simulink model "ConSys_A1"  (Simulink 8.3)
settings: Solver=ode3  StartTime=0.0  StopTime=Time(end)  FixedStep=Ts  RelTol=1e-3
values from neighbouring files (symbols this model uses):
  d = r*h    (= 1.6)    [StartUp_A1.m]
  d0 = d*h    (= 0.0032)    [StartUp_A1.m]
  h = 0.002    [StartUp_A1.m]
  Ka = diag([ 3  20  20  150  355  520])    [StartUp_A1.m]
  Kd = diag([ 3   5  25  100   15 1050])    [StartUp_A1.m]
  Ki = diag([35 555 810 7410 1850 5815])    [StartUp_A1.m]
  Kp = diag([55 180 350 1960  680 4450])    [StartUp_A1.m]
  r = 800    [StartUp_A1.m]
  TD = ss(Atd,Btd,Ctd,Dtd,Ts)    [StartUp_A1.m]
  Ts = 1/200    (= 0.005)    [StartUp_A1.m]
undefined symbols (not defined in the file or in its folder): DiscIntNeverNeededParam
undefined symbols (not defined in the file): ADAMS_cwd, ADAMS_exec, ADAMS_host, ADAMS_init, ADAMS_inputs, ADAMS_outputs, ADAMS_prefix, ADAMS_static, ADAMS_sysdir
libraries: cstblocks x6
(part 3 of 9)

== matlab function A/MATLAB Function 5 ==
  data: q input double; M55 output double; M56 output double
function [M55,M56] = M5(q)
%#codegen
Th1=q(1,1); Th2=q(2,1); Th3=q(3,1);
Th4=q(4,1); Th5=q(5,1); Th6=q(6,1);
M55=2.9736e-6*sin(Th6)^2 + 0.0075895;
M56=(0.5*(sin(Th2 + Th3)*cos(Th5) + cos(Th2 + Th3)*cos(Th4)*sin(Th5))*(0.01294*sin(Th5)*(sin(Th1)*sin(Th4) - 1.0*sin(Th2 + Th3)*cos(Th1)*cos(Th4)) + 0.00023*sin(Th6)*(cos(Th4)*sin(Th1) + sin(Th2 + Th3)*cos(Th1)*sin(Th4)) + 0.00023*cos(Th6)*(cos(Th5)*(sin(Th1)*sin(Th4) - 1.0*sin(Th2 + Th3)*cos(Th1)*cos(Th4)) - 1.0*cos(Th2 + Th3)*cos(Th1)*sin(Th5)) + 0.01294*cos(Th2 + Th3)*cos(Th1)*cos(Th5)) + 0.5*(sin(Th5)*(sin(Th1)*sin(Th4) - 1.0*sin(Th2 + Th3)*cos(Th1)*cos(Th4)) + cos(Th2 + Th3)*cos(Th1)*cos(Th5))*(0.00023*cos(Th6)*(sin(Th2 + Th3)*sin(Th5) - 1.0*cos(Th2 + Th3)*cos(Th4)*cos(Th5)) - 0.01294*sin(Th2 + Th3)*cos(Th5) - 0.01294*cos(Th2 + Th3)*cos(Th4)*sin(Th5) + 0.00023*cos(Th2 + Th3)*sin(Th4)*sin(Th6)))*(0.05206*cos(Th2 + Th3)*sin(Th1)*sin(Th5) + 0.05206*cos(Th1)*cos(Th5)*sin(Th4) - 0.00023*cos(Th2 + Th3)*cos(Th5)*cos(Th6)*sin(Th1) + 0.05206*sin(Th2 + Th3)*cos(Th4)*cos(Th5)*sin(Th1) + 0.00023*cos(Th1)*cos(Th6)*sin(Th4)*sin(Th5) + 0.00023*sin(Th2 + Th3)*cos(Th4)*cos(Th6)*sin(Th1)*sin(Th5)) + (0.000115*cos(Th2 + Th3)*cos(Th6)*sin(Th4) - 0.000115*sin(Th2 + Th3)*sin(Th5)*sin(Th6) + 0.000115*cos(Th2 + Th3)*cos(Th4)*cos(Th5)*sin(Th6))*(0.05206*cos(Th2 + Th3)*cos(Th4)*cos(Th5) - 0.05206*sin(Th2 + Th3)*sin(Th5) + 0.00023*sin(Th2 + Th3)*cos(Th5)*cos(Th6) + 0.00023*cos(Th2 + Th3)*cos(Th4)*cos(Th6)*sin(Th5)) + (sin(Th5)*(cos(Th1)*sin(Th4) + sin(Th2 + Th3)*cos(Th4)*sin(Th1)) - 1.0*cos(Th2 + Th3)*cos(Th5)*sin(Th1))*((cos(Th1)*cos(Th4) - 1.0*sin(Th2 + Th3)*sin(Th1)*sin(Th4))*((0.00104*cos(Th6)*(cos(Th1)*cos(Th4) - 1.0*sin(Th2 + Th3)*sin(Th1)*sin(Th4)) - 0.00104*sin(Th6)*(cos(Th5)*(cos(Th1)*sin(Th4) + sin(Th2 + Th3)*cos(Th4)*sin(Th1)) + cos(Th2 + Th3)*sin(Th1)*sin(Th5)))*(1.0*cos(Th6)*(cos(Th1)*cos(Th4) - 1.0*sin(Th2 + Th3)*sin(Th1)*sin(Th4)) - sin(Th6)*(cos(Th5)*(cos(Th1)*sin(Th4) + sin(Th2 + Th3)*cos(Th4)*sin(Th1)) + cos(Th2 + Th3)*sin(Th1)*sin(Th5))) + (sin(Th5)*(cos(Th1)*sin(Th4) + sin(Th2 + Th3)*cos(Th4)*sin(Th1)) - 1.0*cos(Th2 + Th3)*cos(Th5)*sin(Th1))*(4.0e-6*sin(Th6)*(cos(Th1)*cos(Th4) - 1.0*sin(Th2 + Th3)*sin(Th1)*sin(Th4)) + 4.0e-6*cos(Th6)*(cos(Th5)*(cos(Th1)*sin(Th4) + sin(Th2 + Th3)*cos(Th4)*sin(Th1)) + cos(Th2 + Th3)*sin(Th1)*sin(Th5)) + 0.000116*sin(Th5)*(cos(Th1)*sin(Th4) + sin(Th2 + Th3)*cos(Th4)*sin(Th1)) - 0.000116*cos(Th2 + Th3)*cos(Th5)*sin(Th1)) + (sin(Th6)*(cos(Th1)*cos(Th4) - 1.0*sin(Th2 + Th3)*sin(Th1)*sin(Th4)) + cos(Th6)*(cos(Th5)*(cos(Th1)*sin(Th4) + sin(Th2 + Th3)*cos(Th4)*sin(Th1)) + cos(Th2 + Th3)*sin(Th1)*sin(Th5)))*(0.001043*sin(Th6)*(cos(Th1)*cos(Th4) - 1.0*sin(Th2 + Th3)*sin(Th1)*sin(Th4)) + 0.001043*cos(Th6)*(cos(Th5)*(cos(Th1)*sin(Th4) + sin(Th2 + Th3)*cos(Th4)*sin(Th1)) + cos(Th2 + Th3)*sin(Th1)*sin(Th5)) + 4.0e-6*sin(Th5)*(cos(Th1)*sin(Th4) + sin(Th2 + Th3)*cos(Th4)*sin(Th1)) - 4.0e-6*cos(Th2 + Th3)*cos(Th5)*sin(Th1))) + (cos(Th4)*sin(Th1) + sin(Th2 + Th3)*cos(Th1)*sin(Th4))*((sin(Th6)*(cos(Th1)*cos(Th4) - 1.0*sin(Th2 + Th3)*sin(Th1)*sin(Th4)) + cos(Th6)*(cos(Th5)*(cos(Th1)*sin(Th4) + sin(Th2 + Th3)*cos(Th4)*sin(Th1)) + cos(Th2 + Th3)*sin(Th1)*sin(Th5)))*(4.0e-6*sin(Th5)*(sin(Th1)*sin(Th4) - 1.0*sin(Th2 + Th3)*cos(Th1)*cos(Th4)) + 0.001043*sin(Th6)*(cos(Th4)*sin(Th1) + sin(Th2 + Th3)*cos(Th1)*sin(Th4)) + 0.001043*cos(Th6)*(cos(Th5)*(sin(Th1)*sin(Th4) - 1.0*sin(Th2 + Th3)*cos(Th1)*cos(Th4)) - 1.0*cos(Th2 + Th3)*cos(Th1)*sin(Th5)) + 4.0e-6*cos(Th2 + Th3)*cos(Th1)*cos(Th5)) - (0.00104*sin(Th6)*(cos(Th5)*(sin(Th1)*sin(Th4) - 1.0*sin(Th2 + Th3)*cos(Th1)*cos(Th4)) - 1.0*cos(Th2 + Th3)*cos(Th1)*sin(Th5)) - 0.00104*cos(Th6)*(cos(Th4)*sin(Th1) + sin(Th2 + Th3)*cos(Th1)*sin(Th4)))*(1.0*cos(Th6)*(cos(Th1)*cos(Th4) - 1.0*sin(Th2 + Th3)*sin(Th1)*sin(Th4)) - sin(Th6)*(cos(Th5)*(cos(Th1)*sin(Th4) + sin(Th2 + Th3)*cos(Th4)*sin(Th1)) + cos(Th2 + Th3)*sin(Th1)*sin(Th5))) + (sin(Th5)*(cos(Th1)*sin(Th4) + sin(Th2 + Th3)*cos(Th4)*sin(Th1)) - 1.0*cos(Th2 + Th3)*cos(Th5)*sin(Th1))*(0.000116*sin(Th5)*(sin(Th1)*sin(Th4) - 1.0*sin(Th2 + Th3)*cos(Th1)*cos(Th4)) + 4.0e-6*sin(Th6)*(cos(Th4)*sin(Th1) + sin(Th2 + Th3)*cos(Th1)*sin(Th4)) + 4.0e-6*cos(Th6)*(cos(Th5)*(sin(Th1)*sin(Th4) - 1.0*sin(Th2 + Th3)*cos(Th1)*cos(Th4)) - 1.0*cos(Th2 + Th3)*cos(Th1)*sin(Th5)) + 0.000116*cos(Th2 + Th3)*cos(Th1)*cos(Th5))) + cos(Th2 + Th3)*sin(Th4)*((sin(Th6)*(cos(Th1)*cos(Th4) - 1.0*sin(Th2 + Th3)*sin(Th1)*sin(Th4)) + cos(Th6)*(cos(Th5)*(cos(Th1)*sin(Th4) + sin(Th2 + Th3)*cos(Th4)*sin(Th1)) + cos(Th2 + Th3)*sin(Th1)*sin(Th5)))*(0.001043*cos(Th6)*(sin(Th2 + Th3)*sin(Th5) - 1.0*cos(Th2 + Th3)*cos(Th4)*cos(Th5)) - 4.0e-6*sin(Th2 + Th3)*cos(Th5) - 4.0e-6*cos(Th2 + Th3)*cos(Th4)*sin(Th5) + 0.001043*cos(Th2 + Th3)*sin(Th4)*sin(Th6)) + (sin(Th5)*(cos(Th1)*sin(Th4) + sin(Th2 + Th3)*cos(Th4)*sin(Th1)) - 1.0*cos(Th2 + Th3)*cos(Th5)*sin(Th1))*(4.0e-6*cos(Th6)*(sin(Th2 + Th3)*sin(Th5) - 1.0*cos(Th2 + Th3)*cos(Th4)*cos(Th5)) - 0.000116*sin(Th2 + Th3)*cos(Th5) - 0.000116*cos(Th2 + Th3)*cos(Th4)*sin(Th5) + 4.0e-6*cos(Th2 + Th3)*sin(Th4)*sin(Th6)) - (1.0*cos(Th6)*(cos(Th1)*cos(Th4) - 1.0*sin(Th2 + Th3)*sin(Th1)*sin(Th4)) - sin(Th6)*(cos(Th5)*(cos(Th1)*sin(Th4) + sin(Th2 + Th3)*cos(Th4)*sin(Th1)) + cos(Th2 + Th3)*sin(Th1)*sin(Th5)))*(0.00104*sin(Th6)*(sin(Th2 + Th3)*sin(Th5) - 1.0*cos(Th2 + Th3)*cos(Th4)*cos(Th5)) - 0.00104*cos(Th2 + Th3)*cos(Th6)*sin(Th4)))) - 1.0*(sin(Th2 + Th3)*cos(Th5) + cos(Th2 + Th3)*cos(Th4)*sin(Th5))*((cos(Th4)*sin(Th1) + sin(Th2 + Th3)*cos(Th1)*sin(Th4))*((0.00104*sin(Th6)*(cos(Th5)*(sin(Th1)*sin(Th4) - 1.0*sin(Th2 + Th3)*cos(Th1)*cos(Th4)) - 1.0*cos(Th2 + Th3)*cos(Th1)*sin(Th5)) - 0.00104*cos(Th6)*(cos(Th4)*sin(Th1) + sin(Th2 + Th3)*cos(Th1)*sin(Th4)))*(sin(Th6)*(sin(Th2 + Th3)*sin(Th5) - 1.0*cos(Th2 + Th3)*cos(Th4)*cos(Th5)) - 1.0*cos(Th2 + Th3)*cos(Th6)*sin(Th4)) + (cos(Th6)*(sin(Th2 + Th3)*sin(Th5) - 1.0*cos(Th2 + Th3)*cos(Th4)*cos(Th5)) + cos(Th2 + Th3)*sin(Th4)*sin(Th6))*(4.0e-6*sin(Th5)*(sin(Th1)*sin(Th4) - 1.0*sin(Th2 + Th3)*cos(Th1)*cos(Th4)) + 0.001043*sin(Th6)*(cos(Th4)*sin(Th1) + sin(Th2 + Th3)*cos(Th1)*sin(Th4)) + 0.001043*cos(Th6)*(cos(Th5)*(sin(Th1)*sin(Th4) - 1.0*sin(Th2 + Th3)*cos(Th1)*cos(Th4)) - 1.0*cos(Th2 + Th3)*cos(Th1)*sin(Th5)) + 4.0e-6*cos(Th2 + Th3)*cos(Th1)*cos(Th5)) - 1.0*(sin(Th2 + Th3)*cos(Th5) + cos(Th2 + Th3)*cos(Th4)*sin(Th5))*(0.000116*sin(Th5)*(sin(Th1)*sin(Th4) - 1.0*sin(Th2 + Th3)*cos(Th1)*cos(Th4)) + 4.0e-6*sin(Th6)*(cos(Th4)*sin(Th1) + sin(Th2 + Th3)*cos(Th1)*sin(Th4)) + 4.0e-6*cos(Th6)*(cos(Th5)*(sin(Th1)*sin(Th4) - 1.0*sin(Th2 + Th3)*cos(Th1)*cos(Th4)) - 1.0*cos(Th2 + Th3)*cos(Th1)*sin(Th5)) + 0.000116*cos(Th2 + Th3)*cos(Th1)*cos(Th5))) - (cos(Th1)*cos(Th4) - 1.0*sin(Th2 + Th3)*sin(Th1)*sin(Th4))*((0.00104*cos(Th6)*(cos(Th1)*cos(Th4) - 1.0*sin(Th2 + Th3)*sin(Th1)*sin(Th4)) - 0.00104*sin(Th6)*(cos(Th5)*(cos(Th1)*sin(Th4) + sin(Th2 + Th3)*cos(Th4)*sin(Th1)) + cos(Th2 + Th3)*sin(Th1)*sin(Th5)))*(sin(Th6)*(sin(Th2 + Th3)*sin(Th5) - 1.0*cos(Th2 + Th3)*cos(Th4)*cos(Th5)) - 1.0*cos(Th2 + Th3)*cos(Th6)*sin(Th4)) - (cos(Th6)*(sin(Th2 + Th3)*sin(Th5) - 1.0*cos(Th2 + Th3)*cos(Th4)*cos(Th5)) + cos(Th2 + Th3)*sin(Th4)*sin(Th6))*(0.001043*sin(Th6)*(cos(Th1)*cos(Th4) - 1.0*sin(Th2 + Th3)*sin(Th1)*sin(Th4)) + 0.001043*cos(Th6)*(cos(Th5)*(cos(Th1)*sin(Th4) + sin(Th2 + Th3)*cos(Th4)*sin(Th1)) + cos(Th2 + Th3)*sin(Th1)*sin(Th5)) + 4.0e-6*sin(Th5)*(cos(Th1)*sin(Th4) + sin(Th2 + Th3)*cos(Th4)*sin(Th1)) - 4.0e-6*cos(Th2 + Th3)*cos(Th5)*sin(Th1)) + 1.0*(sin(Th2 + Th3)*cos(Th5) + cos(Th2 + Th3)*cos(Th4)*sin(Th5))*(4.0e-6*sin(Th6)*(cos(Th1)*cos(Th4) - 1.0*sin(Th2 + Th3)*sin(Th1)*sin(Th4)) + 4.0e-6*cos(Th6)*(cos(Th5)*(cos(Th1)*sin(Th4) + sin(Th2 + Th3)*cos(Th4)*sin(Th1)) + cos(Th2 + Th3)*sin(Th1)*sin(Th5)) + 0.000116*sin(Th5)*(cos(Th1)*sin(Th4) + sin(Th2 + Th3)*cos(Th4)*sin(Th1)) - 0.000116*cos(Th2 + Th3)*cos(Th5)*sin(Th1))) + cos(Th2 + Th3)*sin(Th4)*((sin(Th6)*(sin(Th2 + Th3)*sin(Th5) - 1.0*cos(Th2 + Th3)*cos(Th4)*cos(Th5)) - 1.0*cos(Th2 + Th3)*cos(Th6)*sin(Th4))*(0.00104*sin(Th6)*(sin(Th2 + Th3)*sin(Th5) - 1.0*cos(Th2 + Th3)*cos(Th4)*cos(Th5)) - 0.00104*cos(Th2 + Th3)*cos(Th6)*sin(Th4)) - 1.0*(sin(Th2 + Th3)*cos(Th5) + cos(Th2 + Th3)*cos(Th4)*sin(Th5))*(4.0e-6*cos(Th6)*(sin(Th2 + Th3)*sin(Th5) - 1.0*cos(Th2 + Th3)*cos(Th4)*cos(Th5)) - 0.000116*sin(Th2 + Th3)*cos(Th5) - 0.000116*cos(Th2 + Th3)*cos(Th4)*sin(Th5) + 4.0e-6*cos(Th2 + Th3)*sin(Th4)*sin(Th6)) + (cos(Th6)*(sin(Th2 + Th3)*sin(Th5) - 1.0*cos(Th2 + Th3)*cos(Th4)*cos(Th5)) + cos(Th2 + Th3)*sin(Th4)*sin(Th6))*(0.001043*cos(Th6)*(sin(Th2 + Th3)*sin(Th5) - 1.0*cos(Th2 + Th3)*cos(Th4)*cos(Th5)) - 4.0e-6*sin(Th2 + Th3)*cos(Th5) - 4.0e-6*cos(Th2 + Th3)*cos(Th4)*sin(Th5) + 0.001043*cos(Th2 + Th3)*sin(Th4)*sin(Th6)))) + (sin(Th5)*(sin(Th1)*sin(Th4) - 1.0*sin(Th2 + Th3)*cos(Th1)*cos(Th4)) + cos(Th2 + Th3)*cos(Th1)*cos(Th5))*((cos(Th1)*cos(Th4) - 1.0*sin(Th2 + Th3)*sin(Th1)*sin(Th4))*((sin(Th6)*(cos(Th4)*sin(Th1) + sin(Th2 + Th3)*cos(Th1)*sin(Th4)) + cos(Th6)*(cos(Th5)*(sin(Th1)*sin(Th4) - 1.0*sin(Th2 + Th3)*cos(Th1)*cos(Th4)) - 1.0*cos(Th2 + Th3)*cos(Th1)*sin(Th5)))*(0.001043*sin(Th6)*(cos(Th1)*cos(Th4) - 1.0*sin(Th2 + Th3)*sin(Th1)*sin(Th4)) + 0.001043*cos(Th6)*(cos(Th5)*(cos(Th1)*sin(Th4) + sin(Th2 + Th3)*cos(Th4)*sin(Th1)) + cos(Th2 + Th3)*sin(Th1)*sin(Th5)) + 4.0e-6*sin(Th5)*(cos(Th1)*sin(Th4) + sin(Th2 + Th3)*cos(Th4)*sin(Th1)) - 4.0e-6*cos(Th2 + Th3)*cos(Th5)*sin(Th1)) + (sin(Th5)*(sin(Th1)*sin(Th4) - 1.0*sin(Th2 + Th3)*cos(Th1)*cos(Th4)) + cos(Th2 + Th3)*cos(Th1)*cos(Th5))*(4.0e-6*sin(Th6)*(cos(Th1)*cos(Th4) - 1.0*sin(Th2 + Th3)*sin(Th1)*sin(Th4)) + 4.0e-6*cos(Th6)*(cos(Th5)*(cos(Th1)*sin(Th4) + sin(Th2 + Th3)*cos(Th4)*sin(Th1)) + cos(Th2 + Th3)*sin(Th1)*sin(Th5)) + 0.000116*sin(Th5)*(cos(Th1)*sin(Th4) + sin(Th2 + Th3)*cos(Th4)*sin(Th1)) - 0.000116*cos(Th2 + Th3)*cos(Th5)*sin(Th1)) - (0.00104*cos(Th6)*(cos(Th1)*cos(Th4) - 1.0*sin(Th2 + Th3)*sin(Th1)*sin(Th4)) - 0.00104*sin(Th6)*(cos(Th5)*(cos(Th1)*sin(Th4) + sin(Th2 + Th3)*cos(Th4)*sin(Th1)) + cos(Th2 + Th3)*sin(Th1)*sin(Th5)))*(sin(Th6)*(cos(Th5)*(sin(Th1)*sin(Th4) - 1.0*sin(Th2 + Th3)*cos(Th1)*cos(Th4)) - 1.0*cos(Th2 + Th3)*cos(Th1)*sin(Th5)) - 1.0*cos(Th6)*(cos(Th4)*sin(Th1) + sin(Th2 + Th3)*cos(Th1)*sin(Th4)))) + (cos(Th4)*sin(Th1) + sin(Th2 + Th3)*cos(Th1)*sin(Th4))*((0.00104*sin(Th6)*(cos(Th5)*(sin(Th1)*sin(Th4) - 1.0*sin(Th2 + Th3)*cos(Th1)*cos(Th4)) - 1.0*cos(Th2 + Th3)*cos(Th1)*sin(Th5)) - 0.00104*cos(Th6)*(cos(Th4)*sin(Th1) + sin(Th2 + Th3)*cos(Th1)*sin(Th4)))*(sin(Th6)*(cos(Th5)*(sin(Th1)*sin(Th4) - 1.0*sin(Th2 + Th3)*cos(Th1)*cos(Th4)) - 1.0*cos(Th2 + Th3)*cos(Th1)*sin(Th5)) - 1.0*cos(Th6)*(cos(Th4)*sin(Th1) + sin(Th2 + Th3)*cos(Th1)*sin(Th4))) + (sin(Th6)*(cos(Th4)*sin(Th1) + sin(Th2 + Th3)*cos(Th1)*sin(Th4)) + cos(Th6)*(cos(Th5)*(sin(Th1)*sin(Th4) - 1.0*sin(Th2 + Th3)*cos(Th1)*cos(Th4)) - 1.0*cos(Th2 + Th3)*cos(Th1)*sin(Th5)))*(4.0e-6*sin(Th5)*(sin(Th1)*sin(Th4) - 1.0*sin(Th2 + Th3)*cos(Th1)*cos(Th4)) + 0.001043*sin(Th6)*(cos(Th4)*sin(Th1) + sin(Th2 + Th3)*cos(Th1)*sin(Th4)) + 0.001043*cos(Th6)*(cos(Th5)*(sin(Th1)*sin(Th4) - 1.0*sin(Th2 + Th3)*cos(Th1)*cos(Th4)) - 1.0*cos(Th2 + Th3)*cos(Th1)*sin(Th5)) + 4.0e-6*cos(Th2 + Th3)*cos(Th1)*cos(Th5)) + (sin(Th5)*(sin(Th1)*sin(Th4) - 1.0*sin(Th2 + Th3)*cos(Th1)*cos(Th4)) + cos(Th2 + Th3)*cos(Th1)*cos(Th5))*(0.000116*sin(Th5)*(sin(Th1)*sin(Th4) - 1.0*sin(Th2 + Th3)*cos(Th1)*cos(Th4)) + 4.0e-6*sin(Th6)*(cos(Th4)*sin(Th1) + sin(Th2 + Th3)*cos(Th1)*sin(Th4)) + 4.0e-6*cos(Th6)*(cos(Th5)*(sin(Th1)*sin(Th4) - 1.0*sin(Th2 + Th3)*cos(Th1)*cos(Th4)) - 1.0*cos(Th2 + Th3)*cos(Th1)*sin(Th5)) + 0.000116*cos(Th2 + Th3)*cos(Th1)*cos(Th5))) + cos(Th2 + Th3)*sin(Th4)*((0.00104*sin(Th6)*(sin(Th2 + Th3)*sin(Th5) - 1.0*cos(Th2 + Th3)*cos(Th4)*cos(Th5)) - 0.00104*cos(Th2 + Th3)*cos(Th6)*sin(Th4))*(sin(Th6)*(cos(Th5)*(sin(Th1)*sin(Th4) - 1.0*sin(Th2 + Th3)*cos(Th1)*cos(Th4)) - 1.0*cos(Th2 + Th3)*cos(Th1)*sin(Th5)) - 1.0*cos(Th6)*(cos(Th4)*sin(Th1) + sin(Th2 + Th3)*cos(Th1)*sin(Th4))) + (sin(Th6)*(cos(Th4)*sin(Th1) + sin(Th2 + Th3)*cos(Th1)*sin(Th4)) + cos(Th6)*(cos(Th5)*(sin(Th1)*sin(Th4) - 1.0*sin(Th2 + Th3)*cos(Th1)*cos(Th4)) - 1.0*cos(Th2 + Th3)*cos(Th1)*sin(Th5)))*(0.001043*cos(Th6)*(sin(Th2 + Th3)*sin(Th5) - 1.0*cos(Th2 + Th3)*cos(Th4)*cos(Th5)) - 4.0e-6*sin(Th2 + Th3)*cos(Th5) - 4.0e-6*cos(Th2 + Th3)*cos(Th4)*sin(Th5) + 0.001043*cos(Th2 + Th3)*sin(Th4)*sin(Th6)) + (sin(Th5)*(sin(Th1)*sin(Th4) - 1.0*sin(Th2 + Th3)*cos(Th1)*cos(Th4)) + cos(Th2 + Th3)*cos(Th1)*cos(Th5))*(4.0e-6*cos(Th6)*(sin(Th2 + Th3)*sin(Th5) - 1.0*cos(Th2 + Th3)*cos(Th4)*cos(Th5)) - 0.000116*sin(Th2 + Th3)*cos(Th5) - 0.000116*cos(Th2 + Th3)*cos(Th4)*sin(Th5) + 4.0e-6*cos(Th2 + Th3)*sin(Th4)*sin(Th6)))) + (0.5*(sin(Th5)*(cos(Th1)*sin(Th4) + sin(Th2 + Th3)*cos(Th4)*sin(Th1)) - 1.0*cos(Th2 + Th3)*cos(Th5)*sin(Th1))*(0.00023*cos(Th6)*(sin(Th2 + Th3)*sin(Th5) - 1.0*cos(Th2 + Th3)*cos(Th4)*cos(Th5)) - 0.01294*sin(Th2 + Th3)*cos(Th5) - 0.01294*cos(Th2 + Th3)*cos(Th4)*sin(Th5) + 0.00023*cos(Th2 + Th3)*sin(Th4)*sin(Th6)) + 0.5*(sin(Th2 + Th3)*cos(Th5) + cos(Th2 + Th3)*cos(Th4)*sin(Th5))*(0.00023*sin(Th6)*(cos(Th1)*cos(Th4) - 1.0*sin(Th2 + Th3)*sin(Th1)*sin(Th4)) + 0.00023*cos(Th6)*(cos(Th5)*(cos(Th1)*sin(Th4) + sin(Th2 + Th3)*cos(Th4)*sin(Th1)) + cos(Th2 + Th3)*sin(Th1)*sin(Th5)) + 0.01294*sin(Th5)*(cos(Th1)*sin(Th4) + sin(Th2 + Th3)*cos(Th4)*sin(Th1)) - 0.01294*cos(Th2 + Th3)*cos(Th5)*sin(Th1)))*(0.05206*cos(Th2 + Th3)*cos(Th1)*sin(Th5) - 0.05206*cos(Th5)*sin(Th1)*sin(Th4) + 0.05206*sin(Th2 + Th3)*cos(Th1)*cos(Th4)*cos(Th5) - 0.00023*cos(Th6)*sin(Th1)*sin(Th4)*sin(Th5) - 0.00023*cos(Th2 + Th3)*cos(Th1)*cos(Th5)*cos(Th6) + 0.00023*sin(Th2 + Th3)*cos(Th1)*cos(Th4)*cos(Th6)*sin(Th5));
% M61=M16; M31=M13; M41=M14; M51=M15; M21=M12;
end

== matlab function A/MATLAB Function 6 ==
  data: q input double; M66 output double
function M66  = M6(q)
%#codegen
Th1=q(1,1); Th2=q(2,1); Th3=q(3,1);
Th4=q(4,1); Th5=q(5,1); Th6=q(6,1);
M66=0.5*((sin(Th5)*(cos(Th1)*sin(Th4) + sin(Th2 + Th3)*cos(Th4)*sin(Th1)) - 1.0*cos(Th2 + Th3)*cos(Th5)*sin(Th1))*(0.00023*cos(Th6)*(sin(Th2 + Th3)*sin(Th5) - 1.0*cos(Th2 + Th3)*cos(Th4)*cos(Th5)) - 0.01294*sin(Th2 + Th3)*cos(Th5) - 0.01294*cos(Th2 + Th3)*cos(Th4)*sin(Th5) + 0.00023*cos(Th2 + Th3)*sin(Th4)*sin(Th6)) + (sin(Th2 + Th3)*cos(Th5) + cos(Th2 + Th3)*cos(Th4)*sin(Th5))*(0.00023*sin(Th6)*(cos(Th1)*cos(Th4) - 1.0*sin(Th2 + Th3)*sin(Th1)*sin(Th4)) + 0.00023*cos(Th6)*(cos(Th5)*(cos(Th1)*sin(Th4) + sin(Th2 + Th3)*cos(Th4)*sin(Th1)) + cos(Th2 + Th3)*sin(Th1)*sin(Th5)) + 0.01294*sin(Th5)*(cos(Th1)*sin(Th4) + sin(Th2 + Th3)*cos(Th4)*sin(Th1)) - 0.01294*cos(Th2 + Th3)*cos(Th5)*sin(Th1)))^2 + 1.0*(sin(Th2 + Th3)*cos(Th5) + cos(Th2 + Th3)*cos(Th4)*sin(Th5))*((sin(Th5)*(cos(Th1)*sin(Th4) + sin(Th2 + Th3)*cos(Th4)*sin(Th1)) - 1.0*cos(Th2 + Th3)*cos(Th5)*sin(Th1))*((0.00104*cos(Th6)*(cos(Th1)*cos(Th4) - 1.0*sin(Th2 + Th3)*sin(Th1)*sin(Th4)) - 0.00104*sin(Th6)*(cos(Th5)*(cos(Th1)*sin(Th4) + sin(Th2 + Th3)*cos(Th4)*sin(Th1)) + cos(Th2 + Th3)*sin(Th1)*sin(Th5)))*(sin(Th6)*(sin(Th2 + Th3)*sin(Th5) - 1.0*cos(Th2 + Th3)*cos(Th4)*cos(Th5)) - 1.0*cos(Th2 + Th3)*cos(Th6)*sin(Th4)) - (cos(Th6)*(sin(Th2 + Th3)*sin(Th5) - 1.0*cos(Th2 + Th3)*cos(Th4)*cos(Th5)) + cos(Th2 + Th3)*sin(Th4)*sin(Th6))*(0.001043*sin(Th6)*(cos(Th1)*cos(Th4) - 1.0*sin(Th2 + Th3)*sin(Th1)*sin(Th4)) + 0.001043*cos(Th6)*(cos(Th5)*(cos(Th1)*sin(Th4) + sin(Th2 + Th3)*cos(Th4)*sin(Th1)) + cos(Th2 + Th3)*sin(Th1)*sin(Th5)) + 4.0e-6*sin(Th5)*(cos(Th1)*sin(Th4) + sin(Th2 + Th3)*cos(Th4)*sin(Th1)) - 4.0e-6*cos(Th2 + Th3)*cos(Th5)*sin(Th1)) + 1.0*(sin(Th2 + Th3)*cos(Th5) + cos(Th2 + Th3)*cos(Th4)*sin(Th5))*(4.0e-6*sin(Th6)*(cos(Th1)*cos(Th4) - 1.0*sin(Th2 + Th3)*sin(Th1)*sin(Th4)) + 4.0e-6*cos(Th6)*(cos(Th5)*(cos(Th1)*sin(Th4) + sin(Th2 + Th3)*cos(Th4)*sin(Th1)) + cos(Th2 + Th3)*sin(Th1)*sin(Th5)) + 0.000116*sin(Th5)*(cos(Th1)*sin(Th4) + sin(Th2 + Th3)*cos(Th4)*sin(Th1)) - 0.000116*cos(Th2 + Th3)*cos(Th5)*sin(Th1))) + 1.0*(sin(Th2 + Th3)*cos(Th5) + cos(Th2 + Th3)*cos(Th4)*sin(Th5))*((sin(Th6)*(sin(Th2 + Th3)*sin(Th5) - 1.0*cos(Th2 + Th3)*cos(Th4)*cos(Th5)) - 1.0*cos(Th2 + Th3)*cos(Th6)*sin(Th4))*(0.00104*sin(Th6)*(sin(Th2 + Th3)*sin(Th5) - 1.0*cos(Th2 + Th3)*cos(Th4)*cos(Th5)) - 0.00104*cos(Th2 + Th3)*cos(Th6)*sin(Th4)) - 1.0*(sin(Th2 + Th3)*cos(Th5) + cos(Th2 + Th3)*cos(Th4)*sin(Th5))*(4.0e-6*cos(Th6)*(sin(Th2 + Th3)*sin(Th5) - 1.0*cos(Th2 + Th3)*cos(Th4)*cos(Th5)) - 0.000116*sin(Th2 + Th3)*cos(Th5) - 0.000116*cos(Th2 + Th3)*cos(Th4)*sin(Th5) + 4.0e-6*cos(Th2 + Th3)*sin(Th4)*sin(Th6)) + (cos(Th6)*(sin(Th2 + Th3)*sin(Th5) - 1.0*cos(Th2 + Th3)*cos(Th4)*cos(Th5)) + cos(Th2 + Th3)*sin(Th4)*sin(Th6))*(0.001043*cos(Th6)*(sin(Th2 + Th3)*sin(Th5) - 1.0*cos(Th2 + Th3)*cos(Th4)*cos(Th5)) - 4.0e-6*sin(Th2 + Th3)*cos(Th5) - 4.0e-6*cos(Th2 + Th3)*cos(Th4)*sin(Th5) + 0.001043*cos(Th2 + Th3)*sin(Th4)*sin(Th6))) - (sin(Th5)*(sin(Th1)*sin(Th4) - 1.0*sin(Th2 + Th3)*cos(Th1)*cos(Th4)) + cos(Th2 + Th3)*cos(Th1)*cos(Th5))*((0.00104*sin(Th6)*(cos(Th5)*(sin(Th1)*sin(Th4) - 1.0*sin(Th2 + Th3)*cos(Th1)*cos(Th4)) - 1.0*cos(Th2 + Th3)*cos(Th1)*sin(Th5)) - 0.00104*cos(Th6)*(cos(Th4)*sin(Th1) + sin(Th2 + Th3)*cos(Th1)*sin(Th4)))*(sin(Th6)*(sin(Th2 + Th3)*sin(Th5) - 1.0*cos(Th2 + Th3)*cos(Th4)*cos(Th5)) - 1.0*cos(Th2 + Th3)*cos(Th6)*sin(Th4)) + (cos(Th6)*(sin(Th2 + Th3)*sin(Th5) - 1.0*cos(Th2 + Th3)*cos(Th4)*cos(Th5)) + cos(Th2 + Th3)*sin(Th4)*sin(Th6))*(4.0e-6*sin(Th5)*(sin(Th1)*sin(Th4) - 1.0*sin(Th2 + Th3)*cos(Th1)*cos(Th4)) + 0.001043*sin(Th6)*(cos(Th4)*sin(Th1) + sin(Th2 + Th3)*cos(Th1)*sin(Th4)) + 0.001043*cos(Th6)*(cos(Th5)*(sin(Th1)*sin(Th4) - 1.0*sin(Th2 + Th3)*cos(Th1)*cos(Th4)) - 1.0*cos(Th2 + Th3)*cos(Th1)*sin(Th5)) + 4.0e-6*cos(Th2 + Th3)*cos(Th1)*cos(Th5)) - 1.0*(sin(Th2 + Th3)*cos(Th5) + cos(Th2 + Th3)*cos(Th4)*sin(Th5))*(0.000116*sin(Th5)*(sin(Th1)*sin(Th4) - 1.0*sin(Th2 + Th3)*cos(Th1)*cos(Th4)) + 4.0e-6*sin(Th6)*(cos(Th4)*sin(Th1) + sin(Th2 + Th3)*cos(Th1)*sin(Th4)) + 4.0e-6*cos(Th6)*(cos(Th5)*(sin(Th1)*sin(Th4) - 1.0*sin(Th2 + Th3)*cos(Th1)*cos(Th4)) - 1.0*cos(Th2 + Th3)*cos(Th1)*sin(Th5)) + 0.000116*cos(Th2 + Th3)*cos(Th1)*cos(Th5)))) + 0.5*((sin(Th2 + Th3)*cos(Th5) + cos(Th2 + Th3)*cos(Th4)*sin(Th5))*(0.01294*sin(Th5)*(sin(Th1)*sin(Th4) - 1.0*sin(Th2 + Th3)*cos(Th1)*cos(Th4)) + 0.00023*sin(Th6)*(cos(Th4)*sin(Th1) + sin(Th2 + Th3)*cos(Th1)*sin(Th4)) + 0.00023*cos(Th6)*(cos(Th5)*(sin(Th1)*sin(Th4) - 1.0*sin(Th2 + Th3)*cos(Th1)*cos(Th4)) - 1.0*cos(Th2 + Th3)*cos(Th1)*sin(Th5)) + 0.01294*cos(Th2 + Th3)*cos(Th1)*cos(Th5)) + (sin(Th5)*(sin(Th1)*sin(Th4) - 1.0*sin(Th2 + Th3)*cos(Th1)*cos(Th4)) + cos(Th2 + Th3)*cos(Th1)*cos(Th5))*(0.00023*cos(Th6)*(sin(Th2 + Th3)*sin(Th5) - 1.0*cos(Th2 + Th3)*cos(Th4)*cos(Th5)) - 0.01294*sin(Th2 + Th3)*cos(Th5) - 0.01294*cos(Th2 + Th3)*cos(Th4)*sin(Th5) + 0.00023*cos(Th2 + Th3)*sin(Th4)*sin(Th6)))^2 + (sin(Th5)*(cos(Th1)*sin(Th4) + sin(Th2 + Th3)*cos(Th4)*sin(Th1)) - 1.0*cos(Th2 + Th3)*cos(Th5)*sin(Th1))*((sin(Th5)*(sin(Th1)*sin(Th4) - 1.0*sin(Th2 + Th3)*cos(Th1)*cos(Th4)) + cos(Th2 + Th3)*cos(Th1)*cos(Th5))*((sin(Th6)*(cos(Th1)*cos(Th4) - 1.0*sin(Th2 + Th3)*sin(Th1)*sin(Th4)) + cos(Th6)*(cos(Th5)*(cos(Th1)*sin(Th4) + sin(Th2 + Th3)*cos(Th4)*sin(Th1)) + cos(Th2 + Th3)*sin(Th1)*sin(Th5)))*(4.0e-6*sin(Th5)*(sin(Th1)*sin(Th4) - 1.0*sin(Th2 + Th3)*cos(Th1)*cos(Th4)) + 0.001043*sin(Th6)*(cos(Th4)*sin(Th1) + sin(Th2 + Th3)*cos(Th1)*sin(Th4)) + 0.001043*cos(Th6)*(cos(Th5)*(sin(Th1)*sin(Th4) - 1.0*sin(Th2 + Th3)*cos(Th1)*cos(Th4)) - 1.0*cos(Th2 + Th3)*cos(Th1)*sin(Th5)) + 4.0e-6*cos(Th2 + Th3)*cos(Th1)*cos(Th5)) - (0.00104*sin(Th6)*(cos(Th5)*(sin(Th1)*sin(Th4) - 1.0*sin(Th2 + Th3)*cos(Th1)*cos(Th4)) - 1.0*cos(Th2 + Th3)*cos(Th1)*sin(Th5)) - 0.00104*cos(Th6)*(cos(Th4)*sin(Th1) + sin(Th2 + Th3)*cos(Th1)*sin(Th4)))*(1.0*cos(Th6)*(cos(Th1)*cos(Th4) - 1.0*sin(Th2 + Th3)*sin(Th1)*sin(Th4)) - sin(Th6)*(cos(Th5)*(cos(Th1)*sin(Th4) + sin(Th2 + Th3)*cos(Th4)*sin(Th1)) + cos(Th2 + Th3)*sin(Th1)*sin(Th5))) + (sin(Th5)*(cos(Th1)*sin(Th4) + sin(Th2 + Th3)*cos(Th4)*sin(Th1)) - 1.0*cos(Th2 + Th3)*cos(Th5)*sin(Th1))*(0.000116*sin(Th5)*(sin(Th1)*sin(Th4) - 1.0*sin(Th2 + Th3)*cos(Th1)*cos(Th4)) + 4.0e-6*sin(Th6)*(cos(Th4)*sin(Th1) + sin(Th2 + Th3)*cos(Th1)*sin(Th4)) + 4.0e-6*cos(Th6)*(cos(Th5)*(sin(Th1)*sin(Th4) - 1.0*sin(Th2 + Th3)*cos(Th1)*cos(Th4)) - 1.0*cos(Th2 + Th3)*cos(Th1)*sin(Th5)) + 0.000116*cos(Th2 + Th3)*cos(Th1)*cos(Th5))) - 1.0*(sin(Th2 + Th3)*cos(Th5) + cos(Th2 + Th3)*cos(Th4)*sin(Th5))*((sin(Th6)*(cos(Th1)*cos(Th4) - 1.0*sin(Th2 + Th3)*sin(Th1)*sin(Th4)) + cos(Th6)*(cos(Th5)*(cos(Th1)*sin(Th4) + sin(Th2 + Th3)*cos(Th4)*sin(Th1)) + cos(Th2 + Th3)*sin(Th1)*sin(Th5)))*(0.001043*cos(Th6)*(sin(Th2 + Th3)*sin(Th5) - 1.0*cos(Th2 + Th3)*cos(Th4)*cos(Th5)) - 4.0e-6*sin(Th2 + Th3)*cos(Th5) - 4.0e-6*cos(Th2 + Th3)*cos(Th4)*sin(Th5) + 0.001043*cos(Th2 + Th3)*sin(Th4)*sin(Th6)) + (sin(Th5)*(cos(Th1)*sin(Th4) + sin(Th2 + Th3)*cos(Th4)*sin(Th1)) - 1.0*cos(Th2 + Th3)*cos(Th5)*sin(Th1))*(4.0e-6*cos(Th6)*(sin(Th2 + Th3)*sin(Th5) - 1.0*cos(Th2 + Th3)*cos(Th4)*cos(Th5)) - 0.000116*sin(Th2 + Th3)*cos(Th5) - 0.000116*cos(Th2 + Th3)*cos(Th4)*sin(Th5) + 4.0e-6*cos(Th2 + Th3)*sin(Th4)*sin(Th6)) - (1.0*cos(Th6)*(cos(Th1)*cos(Th4) - 1.0*sin(Th2 + Th3)*sin(Th1)*sin(Th4)) - sin(Th6)*(cos(Th5)*(cos(Th1)*sin(Th4) + sin(Th2 + Th3)*cos(Th4)*sin(Th1)) + cos(Th2 + Th3)*sin(Th1)*sin(Th5)))*(0.00104*sin(Th6)*(sin(Th2 + Th3)*sin(Th5) - 1.0*cos(Th2 + Th3)*cos(Th4)*cos(Th5)) - 0.00104*cos(Th2 + Th3)*cos(Th6)*sin(Th4))) + (sin(Th5)*(cos(Th1)*sin(Th4) + sin(Th2 + Th3)*cos(Th4)*sin(Th1)) - 1.0*cos(Th2 + Th3)*cos(Th5)*sin(Th1))*((0.00104*cos(Th6)*(cos(Th1)*cos(Th4) - 1.0*sin(Th2 + Th3)*sin(Th1)*sin(Th4)) - 0.00104*sin(Th6)*(cos(Th5)*(cos(Th1)*sin(Th4) + sin(Th2 + Th3)*cos(Th4)*sin(Th1)) + cos(Th2 + Th3)*sin(Th1)*sin(Th5)))*(1.0*cos(Th6)*(cos(Th1)*cos(Th4) - 1.0*sin(Th2 + Th3)*sin(Th1)*sin(Th4)) - sin(Th6)*(cos(Th5)*(cos(Th1)*sin(Th4) + sin(Th2 + Th3)*cos(Th4)*sin(Th1)) + cos(Th2 + Th3)*sin(Th1)*sin(Th5))) + (sin(Th5)*(cos(Th1)*sin(Th4) + sin(Th2 + Th3)*cos(Th4)*sin(Th1)) - 1.0*cos(Th2 + Th3)*cos(Th5)*sin(Th1))*(4.0e-6*sin(Th6)*(cos(Th1)*cos(Th4) - 1.0*sin(Th2 + Th3)*sin(Th1)*sin(Th4)) + 4.0e-6*cos(Th6)*(cos(Th5)*(cos(Th1)*sin(Th4) + sin(Th2 + Th3)*cos(Th4)*sin(Th1)) + cos(Th2 + Th3)*sin(Th1)*sin(Th5)) + 0.000116*sin(Th5)*(cos(Th1)*sin(Th4) + sin(Th2 + Th3)*cos(Th4)*sin(Th1)) - 0.000116*cos(Th2 + Th3)*cos(Th5)*sin(Th1)) + (sin(Th6)*(cos(Th1)*cos(Th4) - 1.0*sin(Th2 + Th3)*sin(Th1)*sin(Th4)) + cos(Th6)*(cos(Th5)*(cos(Th1)*sin(Th4) + sin(Th2 + Th3)*cos(Th4)*sin(Th1)) + cos(Th2 + Th3)*sin(Th1)*sin(Th5)))*(0.001043*sin(Th6)*(cos(Th1)*cos(Th4) - 1.0*sin(Th2 + Th3)*sin(Th1)*sin(Th4)) + 0.001043*cos(Th6)*(cos(Th5)*(cos(Th1)*sin(Th4) + sin(Th2 + Th3)*cos(Th4)*sin(Th1)) + cos(Th2 + Th3)*sin(Th1)*sin(Th5)) + 4.0e-6*sin(Th5)*(cos(Th1)*sin(Th4) + sin(Th2 + Th3)*cos(Th4)*sin(Th1)) - 4.0e-6*cos(Th2 + Th3)*cos(Th5)*sin(Th1)))) + (sin(Th5)*(sin(Th1)*sin(Th4) - 1.0*sin(Th2 + Th3)*cos(Th1)*cos(Th4)) + cos(Th2 + Th3)*cos(Th1)*cos(Th5))*((sin(Th5)*(sin(Th1)*sin(Th4) - 1.0*sin(Th2 + Th3)*cos(Th1)*cos(Th4)) + cos(Th2 + Th3)*cos(Th1)*cos(Th5))*((0.00104*sin(Th6)*(cos(Th5)*(sin(Th1)*sin(Th4) - 1.0*sin(Th2 + Th3)*cos(Th1)*cos(Th4)) - 1.0*cos(Th2 + Th3)*cos(Th1)*sin(Th5)) - 0.00104*cos(Th6)*(cos(Th4)*sin(Th1) + sin(Th2 + Th3)*cos(Th1)*sin(Th4)))*(sin(Th6)*(cos(Th5)*(sin(Th1)*sin(Th4) - 1.0*sin(Th2 + Th3)*cos(Th1)*cos(Th4)) - 1.0*cos(Th2 + Th3)*cos(Th1)*sin(Th5)) - 1.0*cos(Th6)*(cos(Th4)*sin(Th1) + sin(Th2 + Th3)*cos(Th1)*sin(Th4))) + (sin(Th6)*(cos(Th4)*sin(Th1) + sin(Th2 + Th3)*cos(Th1)*sin(Th4)) + cos(Th6)*(cos(Th5)*(sin(Th1)*sin(Th4) - 1.0*sin(Th2 + Th3)*cos(Th1)*cos(Th4)) - 1.0*cos(Th2 + Th3)*cos(Th1)*sin(Th5)))*(4.0e-6*sin(Th5)*(sin(Th1)*sin(Th4) - 1.0*sin(Th2 + Th3)*cos(Th1)*cos(Th4)) + 0.001043*sin(Th6)*(cos(Th4)*sin(Th1) + sin(Th2 + Th3)*cos(Th1)*sin(Th4)) + 0.001043*cos(Th6)*(cos(Th5)*(sin(Th1)*sin(Th4) - 1.0*sin(Th2 + Th3)*cos(Th1)*cos(Th4)) - 1.0*cos(Th2 + Th3)*cos(Th1)*sin(Th5)) + 4.0e-6*cos(Th2 + Th3)*cos(Th1)*cos(Th5)) + (sin(Th5)*(sin(Th1)*sin(Th4) - 1.0*sin(Th2 + Th3)*cos(Th1)*cos(Th4)) + cos(Th2 + Th3)*cos(Th1)*cos(Th5))*(0.000116*sin(Th5)*(sin(Th1)*sin(Th4) - 1.0*sin(Th2 + Th3)*cos(Th1)*cos(Th4)) + 4.0e-6*sin(Th6)*(cos(Th4)*sin(Th1) + sin(Th2 + Th3)*cos(Th1)*sin(Th4)) + 4.0e-6*cos(Th6)*(cos(Th5)*(sin(Th1)*sin(Th4) - 1.0*sin(Th2 + Th3)*cos(Th1)*cos(Th4)) - 1.0*cos(Th2 + Th3)*cos(Th1)*sin(Th5)) + 0.000116*cos(Th2 + Th3)*cos(Th1)*cos(Th5))) + (sin(Th5)*(cos(Th1)*sin(Th4) + sin(Th2 + Th3)*cos(Th4)*sin(Th1)) - 1.0*cos(Th2 + Th3)*cos(Th5)*sin(Th1))*((sin(Th6)*(cos(Th4)*sin(Th1) + sin(Th2 + Th3)*cos(Th1)*sin(Th4)) + cos(Th6)*(cos(Th5)*(sin(Th1)*sin(Th4) - 1.0*sin(Th2 + Th3)*cos(Th1)*cos(Th4)) - 1.0*cos(Th2 + Th3)*cos(Th1)*sin(Th5)))*(0.001043*sin(Th6)*(cos(Th1)*cos(Th4) - 1.0*sin(Th2 + Th3)*sin(Th1)*sin(Th4)) + 0.001043*cos(Th6)*(cos(Th5)*(cos(Th1)*sin(Th4) + sin(Th2 + Th3)*cos(Th4)*sin(Th1)) + cos(Th2 + Th3)*sin(Th1)*sin(Th5)) + 4.0e-6*sin(Th5)*(cos(Th1)*sin(Th4) + sin(Th2 + Th3)*cos(Th4)*sin(Th1)) - 4.0e-6*cos(Th2 + Th3)*cos(Th5)*sin(Th1)) + (sin(Th5)*(sin(Th1)*sin(Th4) - 1.0*sin(Th2 + Th3)*cos(Th1)*cos(Th4)) + cos(Th2 + Th3)*cos(Th1)*cos(Th5))*(4.0e-6*sin(Th6)*(cos(Th1)*cos(Th4) - 1.0*sin(Th2 + Th3)*sin(Th1)*sin(Th4)) + 4.0e-6*cos(Th6)*(cos(Th5)*(cos(Th1)*sin(Th4) + sin(Th2 + Th3)*cos(Th4)*sin(Th1)) + cos(Th2 + Th3)*sin(Th1)*sin(Th5)) + 0.000116*sin(Th5)*(cos(Th1)*sin(Th4) + sin(Th2 + Th3)*cos(Th4)*sin(Th1)) - 0.000116*cos(Th2 + Th3)*cos(Th5)*sin(Th1)) - (0.00104*cos(Th6)*(cos(Th1)*cos(Th4) - 1.0*sin(Th2 + Th3)*sin(Th1)*sin(Th4)) - 0.00104*sin(Th6)*(cos(Th5)*(cos(Th1)*sin(Th4) + sin(Th2 + Th3)*cos(Th4)*sin(Th1)) + cos(Th2 + Th3)*sin(Th1)*sin(Th5)))*(sin(Th6)*(cos(Th5)*(sin(Th1)*sin(Th4) - 1.0*sin(Th2 + Th3)*cos(Th1)*cos(Th4)) - 1.0*cos(Th2 + Th3)*cos(Th1)*sin(Th5)) - 1.0*cos(Th6)*(cos(Th4)*sin(Th1) + sin(Th2 + Th3)*cos(Th1)*sin(Th4)))) - 1.0*(sin(Th2 + Th3)*cos(Th5) + cos(Th2 + Th3)*cos(Th4)*sin(Th5))*((0.00104*sin(Th6)*(sin(Th2 + Th3)*sin(Th5) - 1.0*cos(Th2 + Th3)*cos(Th4)*cos(Th5)) - 0.00104*cos(Th2 + Th3)*cos(Th6)*sin(Th4))*(sin(Th6)*(cos(Th5)*(sin(Th1)*sin(Th4) - 1.0*sin(Th2 + Th3)*cos(Th1)*cos(Th4)) - 1.0*cos(Th2 + Th3)*cos(Th1)*sin(Th5)) - 1.0*cos(Th6)*(cos(Th4)*sin(Th1) + sin(Th2 + Th3)*cos(Th1)*sin(Th4))) + (sin(Th6)*(cos(Th4)*sin(Th1) + sin(Th2 + Th3)*cos(Th1)*sin(Th4)) + cos(Th6)*(cos(Th5)*(sin(Th1)*sin(Th4) - 1.0*sin(Th2 + Th3)*cos(Th1)*cos(Th4)) - 1.0*cos(Th2 + Th3)*cos(Th1)*sin(Th5)))*(0.001043*cos(Th6)*(sin(Th2 + Th3)*sin(Th5) - 1.0*cos(Th2 + Th3)*cos(Th4)*cos(Th5)) - 4.0e-6*sin(Th2 + Th3)*cos(Th5) - 4.0e-6*cos(Th2 + Th3)*cos(Th4)*sin(Th5) + 0.001043*cos(Th2 + Th3)*sin(Th4)*sin(Th6)) + (sin(Th5)*(sin(Th1)*sin(Th4) - 1.0*sin(Th2 + Th3)*cos(Th1)*cos(Th4)) + cos(Th2 + Th3)*cos(Th1)*cos(Th5))*(4.0e-6*cos(Th6)*(sin(Th2 + Th3)*sin(Th5) - 1.0*cos(Th2 + Th3)*cos(Th4)*cos(Th5)) - 0.000116*sin(Th2 + Th3)*cos(Th5) - 0.000116*cos(Th2 + Th3)*cos(Th4)*sin(Th5) + 4.0e-6*cos(Th2 + Th3)*sin(Th4)*sin(Th6)))) + 0.5*(0.00023*cos(Th2 + Th3)*cos(Th6)*sin(Th4) - 0.00023*sin(Th2 + Th3)*sin(Th5)*sin(Th6) + 0.00023*cos(Th2 + Th3)*cos(Th4)*cos(Th5)*sin(Th6))^2;
end

== matlab function A1/MATLAB Function 1 ==
  data: q input double; G11 output double; G21 output double; G31 output double; G41 output double; G51 output double; G61 output double
function [G11,G21,G31,G41,G51,G61] = G(q)
%#codegen
Th1=q(1,1); Th2=q(2,1); Th3=q(3,1);
Th4=q(4,1); Th5=q(5,1); Th6=q(6,1);
G11=0;
G21=3.1202*cos(Th2)*cos(Th3) - 140.4*sin(Th2) - 2.3855*cos(Th2) + 0.1571*cos(Th2)*sin(Th3) + 0.1571*cos(Th3)*sin(Th2) - 3.1202*sin(Th2)*sin(Th3) + 0.24036*cos(Th2)*cos(Th3)*cos(Th5) - 0.00019613*cos(Th2)*cos(Th3)*sin(Th5) - 0.0060801*cos(Th2)*sin(Th3)*sin(Th4) - 0.0060801*cos(Th3)*sin(Th2)*sin(Th4) - 0.24036*cos(Th5)*sin(Th2)*sin(Th3) + 0.00019613*sin(Th2)*sin(Th3)*sin(Th5) - 0.00019613*cos(Th2)*cos(Th4)*cos(Th5)*sin(Th3) - 0.00019613*cos(Th3)*cos(Th4)*cos(Th5)*sin(Th2) + 0.0011278*cos(Th2)*cos(Th3)*cos(Th6)*sin(Th5) - 0.24036*cos(Th2)*cos(Th4)*sin(Th3)*sin(Th5) - 0.24036*cos(Th3)*cos(Th4)*sin(Th2)*sin(Th5) - 0.0011278*cos(Th2)*sin(Th3)*sin(Th4)*sin(Th6) - 0.0011278*cos(Th3)*sin(Th2)*sin(Th4)*sin(Th6) - 0.0011278*cos(Th6)*sin(Th2)*sin(Th3)*sin(Th5) + 0.0011278*cos(Th2)*cos(Th4)*cos(Th5)*cos(Th6)*sin(Th3) + 0.0011278*cos(Th3)*cos(Th4)*cos(Th5)*cos(Th6)*sin(Th2);
G31=3.1202*cos(Th2)*cos(Th3) + 0.1571*cos(Th2)*sin(Th3) + 0.1571*cos(Th3)*sin(Th2) - 3.1202*sin(Th2)*sin(Th3) + 0.24036*cos(Th2)*cos(Th3)*cos(Th5) - 0.00019613*cos(Th2)*cos(Th3)*sin(Th5) - 0.0060801*cos(Th2)*sin(Th3)*sin(Th4) - 0.0060801*cos(Th3)*sin(Th2)*sin(Th4) - 0.24036*cos(Th5)*sin(Th2)*sin(Th3) + 0.00019613*sin(Th2)*sin(Th3)*sin(Th5) - 0.00019613*cos(Th2)*cos(Th4)*cos(Th5)*sin(Th3) - 0.00019613*cos(Th3)*cos(Th4)*cos(Th5)*sin(Th2) + 0.0011278*cos(Th2)*cos(Th3)*cos(Th6)*sin(Th5) - 0.24036*cos(Th2)*cos(Th4)*sin(Th3)*sin(Th5) - 0.24036*cos(Th3)*cos(Th4)*sin(Th2)*sin(Th5) - 0.0011278*cos(Th2)*sin(Th3)*sin(Th4)*sin(Th6) - 0.0011278*cos(Th3)*sin(Th2)*sin(Th4)*sin(Th6) - 0.0011278*cos(Th6)*sin(Th2)*sin(Th3)*sin(Th5) + 0.0011278*cos(Th2)*cos(Th4)*cos(Th5)*cos(Th6)*sin(Th3) + 0.0011278*cos(Th3)*cos(Th4)*cos(Th5)*cos(Th6)*sin(Th2);
G41=0.000049033*cos(Th2 + Th3)*(124.0*cos(Th4) - 4.0*cos(Th5)*sin(Th4) + 23.0*cos(Th4)*sin(Th6) - 4902.0*sin(Th4)*sin(Th5) + 23.0*cos(Th5)*cos(Th6)*sin(Th4));
G51=0.24036*cos(Th2 + Th3)*cos(Th4)*cos(Th5) - 0.24036*sin(Th2 + Th3)*sin(Th5) - 0.00019613*sin(Th2 + Th3)*cos(Th5) - 0.00019613*cos(Th2 + Th3)*cos(Th4)*sin(Th5) + 0.0011278*sin(Th2 + Th3)*cos(Th5)*cos(Th6) + 0.0011278*cos(Th2 + Th3)*cos(Th4)*cos(Th6)*sin(Th5);
G61=0.0011278*cos(Th2 + Th3)*cos(Th6)*sin(Th4) - 0.0011278*sin(Th2 + Th3)*sin(Th5)*sin(Th6) + 0.0011278*cos(Th2 + Th3)*cos(Th4)*cos(Th5)*sin(Th6);
end
